simulink model "SubLab"  (Simulink 7.6)
settings: Solver=ode45  StartTime=0.0  StopTime=30.0  RelTol=1e-3
values from neighbouring files (symbols this model uses):
  b2 = 0.1    [SubLabParameters.m]
  denom = [a b c d e]    [SubLabParameters.m]
  k2 = 49    [SubLabParameters.m]
  m2 = 1    [SubLabParameters.m]
settings Model: Creator=m134506  LastModifiedBy=m134506
settings DataIOCC: LimitDataPoints=off  TimeSaveName=t  Refine=1000

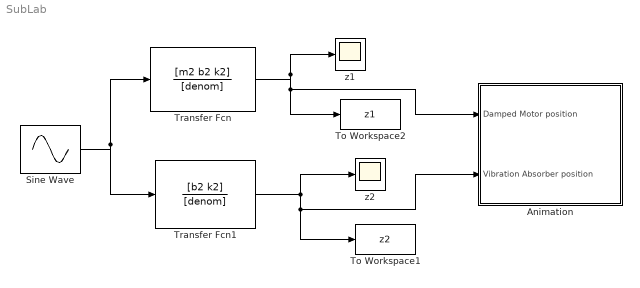
== system SubLab ==
  Animation : Subsystem
  Sine Wave : Sin  Frequency=7  SampleTime=0
  To Workspace1 : ToWorkspace  VariableName=z2  SampleTime=-1  SaveFormat=Array
  To Workspace2 : ToWorkspace  VariableName=z1  SampleTime=-1  SaveFormat=Array
  Transfer Fcn : TransferFcn  Numerator=[m2 b2 k2]  Denominator=[denom]
  Transfer Fcn1 : TransferFcn  Numerator=[b2 k2]  Denominator=[denom]
  z1 : Scope
  z2 : Scope
  wires:
  Transfer Fcn/1 -> z1/1, To Workspace2/1, Animation/1(Damped Motor position)
  Transfer Fcn1/1 -> z2/1, To Workspace1/1, Animation/2(Vibration Absorber position)
  Sine Wave/1 -> Transfer Fcn/1, Transfer Fcn1/1

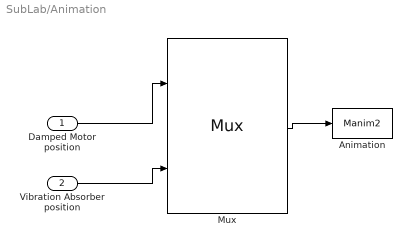
== system SubLab/Animation ==
  Damped Motor position : Inport
  Vibration Absorber position : Inport  Port=2
  Animation : S-Function  FunctionName=Manim2  EnableBusSupport=off
  Mux : Mux  Inputs=2
  wires:
  Damped Motor position/1 -> Mux/1
  Vibration Absorber position/1 -> Mux/2
  Mux/1 -> Animation/1
